simulink model "Timer"  (Simulink 7.4)
settings: Solver=ode1  SolverMode=SingleTasking  StartTime=0.0  StopTime=inf  FixedStep=0.01  MaxStep=0.02  RelTol=1e-3  AbsTol=1e-6
libraries: simulink x2
CloseFcn:
  | rtwprivate ssgencode ModelCloseRequest MC_AD
settings Model: Creator=Admin  LastModifiedBy=fw  SimulationMode=external
settings ConfigSet: Description=rtmc9s12target_R2009b
settings DataIOCC: LimitDataPoints=off  SaveOutput=off  SaveTime=off  SignalLoggingName=sigsOut
settings OptimizationCC: BlockReduction=off  BooleanDataType=off  InitFltsAndDblsToZero=on  OptimizeModelRefInitCode=on  LifeSpan=1
settings DebuggingCC: SaveWithParameterizedLinksMsg=none  SignalResolutionControl=TryResolveAllWithWarning  SolverPrmCheckMsg=none  MultiTaskDSMMsg=warning  MultiTaskCondExecSysMsg=none  StrictBusMsg=None
settings HardwareCC: ProdBitPerInt=16  ProdEndianess=BigEndian  ProdWordSize=16  ProdHWDeviceType=Motorola HC12
settings RTWCC: SystemTargetFile=mc9s12.tlc  GenerateMakefile=off  TemplateMakefile=mc9s12.tmf  ProcessScript=mc9s12_make_rtw_hook  IncludeERTFirstTime=on
settings CodeAppCC: IgnoreCustomStorageClasses=off
settings STFCustomTargetCC: TargetFcnLib=ansi_tfl_tmw.mat  ModelReferenceCompliant=off  IncludeMdlTerminateFcn=off  ERTCustomFileBanners=on  SupportNonInlinedSFcns=off  CPPClassGenCompliant=on  SystemTargetFile=mc9s12.tlc
settings ERTTargetCC: TargetFcnLib=ansi_tfl_tmw.mat  MultiwordLength=2048  ModelReferenceCompliant=off  ParMdlRefBuildCompliant=off  CompOptLevelCompliant=off  IncludeMdlTerminateFcn=off  CombineOutputUpdateFcns=off  ERTFirstTimeCompliant=off  SupportContinuousTime=on  ModelStepFunctionPrototypeControlCompliant=off  ExtMode=on  ExtModeMexFile=ext_serial_mc9s12_comm  ExtModeMexArgs=1,2,115200  InlinedParameterPlacement=NonHierarchical  ERTCustomFileTemplate=mc9s12_file_process.tlc  GRTInterface=on  ConvertIfToSwitch=off
settings CustomProperty: DataType=RTWOptions_EnumType_C__Users_fw__SVN_rtmc9s12-target_trunk_rtmc9s12_CW_R2009b_bin_mc9s12_1mc9s12_TargetBoard  Value=Dragon12Plus
settings EnumStrPairs: String=Dragon12

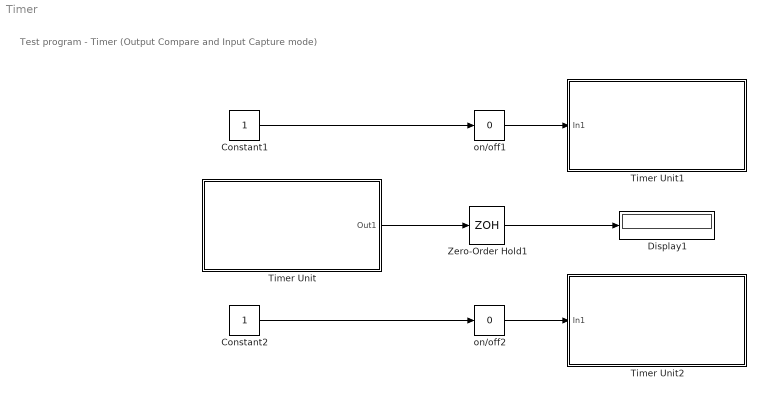
== system Timer ==
  note: Test program - Timer (Output Compare and Input Capture mode)
  Constant1 : Constant  OutDataType=sfix(16)  OutScaling=2^0
  Constant2 : Constant  OutDataType=sfix(16)  OutScaling=2^0
  Display1 : Display
  Timer Unit : Subsystem  Tag=mcTarget_timer  mask{timerChannel=Channel 3, timerMode=Input Capture, timerPeriod=0.3, sampletime=0.1}
      mask prompts: timerChannel "Timer channel"; timerMode "Timer mode"; timerPeriod "Timer base period (seconds)"; sampletime "Sample time"
      mask init:
      | if(timerMode == 1)
      | 	% OC
      | 	timerPeriodTypestr = 'Period:';
      | else
      | 	% IC
      | 	timerPeriodTypestr = 'Measurement intvl:';
      | end
      | 
      | [timerChannelstr, timerModestr, timerPeriodstr, ECTResolutionstr] = mbc_timer(timerChannel, timerMode, timerPeriod, sampletime);
      | 
      | % future extension: allow for output port / pin selection
      | % this hasn't been implemented yet, as it would require the 
      | % interrupt service handlers to be configured by TLC
      | % fw-09-06
      | %
      | % the following code assumes that timerOCport and timerOCpin have been defined similarly to what's done in mbc_ditaloutput.m
      | % the function also returns two more parameters (timerPORTstr, timerPINstr)
      | % these can be used in the Icon page. Replace that line by the following:
      | % fprintf('Channel: %s\nMode: %s\n%sPeriod: %s\nResolution: %s', timerChannelstr, timerModestr, timerOptPORTstr, timerPeriodstr, ECTResolutionstr)
      | % 
      | % [timerChannelstr, timerModestr, timerPORTstr, timerPINstr, timerPeriodstr, ECTResolutionstr] = mbc_timer(timerChannel, timerMode, timerOCport, timerOCpin, timerPeriod, sampletime);
      | % 
      | % if(timerMode == 1)
      | % 	% OC -> display port / pin
      | % 	timerOptPORTstr = ['Toggle: ' timerPORTstr ', Pin(s): ' timerPINstr '\n'];
      | % else
      | % 	% IC -> don't display port / pin
      | % 	timerOptPORTstr = '';
      | % end
      mask Help: web('timer_sfcn_9S12.html');
      mask StyleString: popup(Channel 0|Channel 1|Channel 2|Channel 3|Channel 4|Channel 5|Channel 6),popup(Output Compare|Input Capture),edit,edit
      mask Display: fprintf('Channel: %s\nMode: %s\nPeriod: %s\nResolution: %s', timerChannelstr, timerModestr, timerPeriodstr, ECTResolutionstr)
  Timer Unit1 : Subsystem  Tag=mcTarget_timer  mask{timerChannel=Channel 1, timerMode=Output Compare, timerPeriod=0.3, sampletime=0.1}
      mask prompts: timerChannel "Timer channel"; timerMode "Timer mode"; timerPeriod "Timer base period (seconds)"; sampletime "Sample time"
      mask init: same as Timer/Timer Unit
      mask Help: web('timer_sfcn_9S12.html');
      mask StyleString: popup(Channel 0|Channel 1|Channel 2|Channel 3|Channel 4|Channel 5|Channel 6),popup(Output Compare|Input Capture),edit,edit
      mask Display: fprintf('Channel: %s\nMode: %s\nPeriod: %s\nResolution: %s', timerChannelstr, timerModestr, timerPeriodstr, ECTResolutionstr)
  Timer Unit2 : Subsystem  Tag=mcTarget_timer  mask{timerChannel=Channel 2, timerMode=Output Compare, timerPeriod=0.0001, sampletime=0.1}
      mask prompts: timerChannel "Timer channel"; timerMode "Timer mode"; timerPeriod "Timer base period (seconds)"; sampletime "Sample time"
      mask init: same as Timer/Timer Unit
      mask Help: web('timer_sfcn_9S12.html');
      mask StyleString: popup(Channel 0|Channel 1|Channel 2|Channel 3|Channel 4|Channel 5|Channel 6),popup(Output Compare|Input Capture),edit,edit
      mask Display: fprintf('Channel: %s\nMode: %s\nPeriod: %s\nResolution: %s', timerChannelstr, timerModestr, timerPeriodstr, ECTResolutionstr)
  Zero-Order Hold1 : ZeroOrderHold  SampleTime=0.1
  on/off1 : simulink/Math Operations/Slider Gain  SystemSampleTime=-1  low=0  gain=0  high=1
  on/off2 : simulink/Math Operations/Slider Gain  SystemSampleTime=-1  low=0  gain=0  high=1
  wires:
  Zero-Order Hold1/1 -> Display1/1
  Timer Unit/1(Out1) -> Zero-Order Hold1/1
  Constant1/1 -> on/off1/1
  on/off1/1 -> Timer Unit1/1(In1)
  Constant2/1 -> on/off2/1
  on/off2/1 -> Timer Unit2/1(In1)

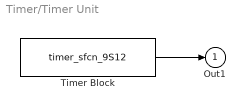
== system Timer/Timer Unit ==
  Timer Block : S-Function  Tag=mcTarget_timer  FunctionName=timer_sfcn_9S12  Parameters=sampletime, timerMode  EnableBusSupport=off
  Out1 : Outport
  wires:
  Timer Block/1 -> Out1/1

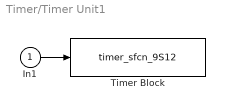
== system Timer/Timer Unit1 ==
  In1 : Inport  OutDataType=sfix(16)  OutScaling=2^0
  Timer Block : S-Function  Tag=mcTarget_timer  FunctionName=timer_sfcn_9S12  Parameters=sampletime, timerMode  EnableBusSupport=off
  wires:
  In1/1 -> Timer Block/1

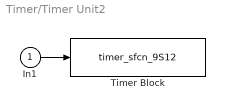
== system Timer/Timer Unit2 ==
  In1 : Inport  OutDataType=sfix(16)  OutScaling=2^0
  Timer Block : S-Function  Tag=mcTarget_timer  FunctionName=timer_sfcn_9S12  Parameters=sampletime, timerMode  EnableBusSupport=off
  wires:
  In1/1 -> Timer Block/1
